simulink library "lapCounter_ul"  (R2018a)
settings: Solver=VariableStepAuto  StartTime=0.0  StopTime=10.0  RelTol=1e-3
libraries: simulink x2
settings Model: Creator=mcobb  LastModifiedBy=mcobb

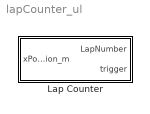
== system lapCounter_ul ==
  Lap Counter : Subsystem

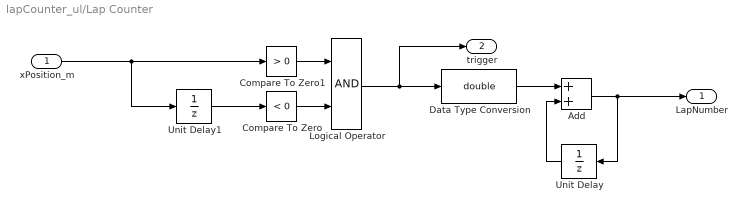
== system lapCounter_ul/Lap Counter ==
  xPosition_m : Inport
  Add : Sum
  Compare To Zero : simulink/Logic and Bit Operations/Compare To Zero  relop=<  OutDataTypeStr=boolean
  Compare To Zero1 : simulink/Logic and Bit Operations/Compare To Zero  relop=>  OutDataTypeStr=boolean
  Data Type Conversion : DataTypeConversion  OutDataTypeStr=double
  Logical Operator : Logic  AllPortsSameDT=off  OutDataTypeStr=boolean
  Unit Delay : UnitDelay  InitialCondition=1  SampleTime=-1
  Unit Delay1 : UnitDelay  SampleTime=-1
  LapNumber : Outport
  trigger : Outport  Port=2
  wires:
  Add/1 -> Unit Delay/1, LapNumber/1
  Logical Operator/1 -> trigger/1, Data Type Conversion/1
  Unit Delay/1 -> Add/2
  xPosition_m/1 -> Compare To Zero1/1, Unit Delay1/1
  Unit Delay1/1 -> Compare To Zero/1
  Compare To Zero1/1 -> Logical Operator/1
  Compare To Zero/1 -> Logical Operator/2
  Data Type Conversion/1 -> Add/1
